simulink model "Model_Guido_v4_2020a"  (R2020a)
settings: Solver=FixedStepAuto  StartTime=0.0  StopTime=10  RelTol=1e-3
undefined symbols (not defined in the file): Bvx, Bvy, Bw, Cvx, Cvy, Cw, d, DiscIntNeverNeededParam, J, K_fsfb, K_int, Kt, l, M, r, Ti, Ts
libraries: simulink x1
settings Model: Creator=User  LastModifiedBy=User
settings SolverCC: ZeroCrossControl=EnableAll  ZeroCrossAlgorithm=Adaptive
settings DebuggingCC: IgnoredZcDiagnostic=none

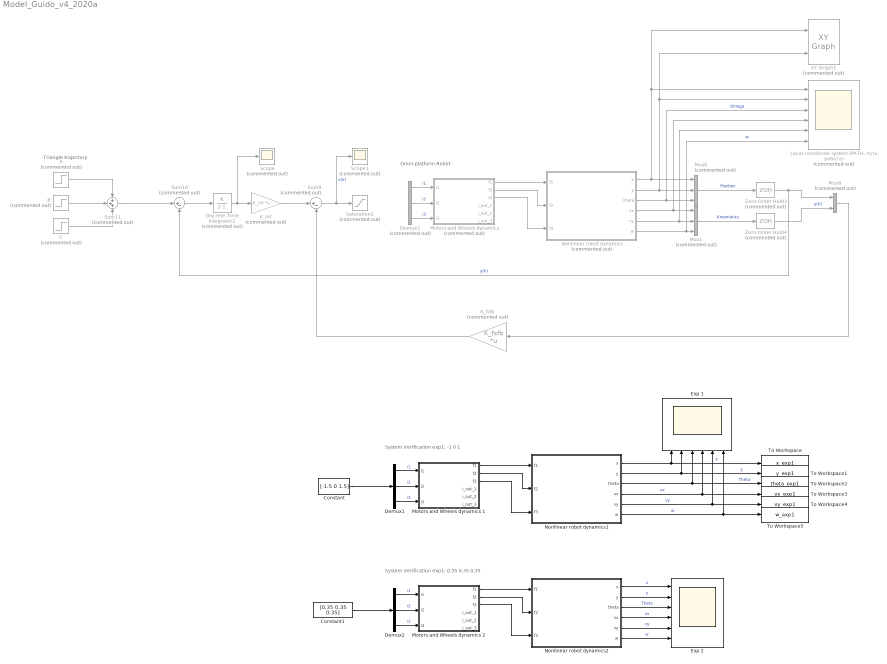
== system Model_Guido_v4_2020a ==
  note: Omni-platform Robot
  note: Triangle trajectory
  note: System Verification exp1: -1 0 1
  note: System Verification exp1: 0.35 0.35 0.35
  A : Step  Commented=on  Time=0  Before=[1 0.5 pi/2]  After=[0.5 -sqrt(3)/2 1]  SampleTime=Ts
  B : Step  Commented=on  Time=6  Before=[0 0 0]  After=[-1 0 1]  SampleTime=Ts
  C : Step  Commented=on  Time=12  Before=[0 0 0]  After=[0.5 sqrt(3)/2 0]  SampleTime=Ts
  Constant : Constant  Value=[-1.5 0 1.5]  SampleTime=0.0866
  Constant1 : Constant  Value=[0.35 0.35 0.35]  SampleTime=0.02
  Demux1 : Demux  Outputs=3
  Demux2 : Demux  Outputs=3
  Demux3 : Demux  Commented=on  Outputs=3
  Discrete-Time Integrator2 : DiscreteIntegrator  Commented=on  IntegratorMethod=Accumulation: Forward Euler  InitialCondition=[ 0 0 0]  SampleTime=Ts  ICPrevOutput=DiscIntNeverNeededParam  ICPrevScaledInput=DiscIntNeverNeededParam
  Exp 1 : Scope  NumInputPorts=6
  Exp 2 : Scope  NumInputPorts=6
  K_fsfb : Gain  Commented=on  Gain=K_fsfb  Multiplication=Matrix(K*u) (u vector)
  K_int : Gain  Commented=on  Gain=K_int  Multiplication=Matrix(K*u) (u vector)
  "Local coordinate system (PATH, путь робота)" : Scope  Commented=on  NumInputPorts=6
  "Motors and Wheels dynamics " : Subsystem  Commented=on
  Motors and Wheels dynamics 1 : Subsystem
  Motors and Wheels dynamics 2 : Subsystem
  Mux1 : Mux  Commented=on  Inputs=3
  Mux6 : Mux  Commented=on  Inputs=3
  Mux8 : Mux  Commented=on  Inputs=2
  Nonlinear robot dynamics : Subsystem  Commented=on
  Nonlinear robot dynamics1 : Subsystem
  Nonlinear robot dynamics2 : Subsystem
  Saturation2 : Saturate  Commented=on  UpperLimit=1  LowerLimit=-1
  Scope : Scope  Commented=on
  Scope1 : Scope  Commented=on
  Sum10 : Sum  Commented=on  Inputs=|+-
  Sum11 : Sum  Commented=on  Inputs=+++
  Sum9 : Sum  Commented=on  Inputs=|+-
  To Workspace : ToWorkspace  VariableName=x_exp1  SampleTime=-1
      settings: Save2DSignal=2-D array (concatenate along first dimension)
  To Workspace1 : ToWorkspace  VariableName=y_exp1  SaveFormat=Timeseries  SampleTime=-1
  To Workspace2 : ToWorkspace  VariableName=theta_exp1  SaveFormat=Timeseries  SampleTime=-1
  To Workspace3 : ToWorkspace  VariableName=vx_exp1  SaveFormat=Timeseries  SampleTime=-1
  To Workspace4 : ToWorkspace  VariableName=vy_exp1  SaveFormat=Timeseries  SampleTime=-1
  To Workspace5 : ToWorkspace  VariableName=w_exp1  SaveFormat=Timeseries  SampleTime=-1
  XY Graph1 : simulink/Sinks/XY Graph  Commented=on  xmin=-1  xmax=1  ymin=-1  ymax=1  st=-1
  Zero-Order Hold3 : ZeroOrderHold  Commented=on  SampleTime=Ts
  Zero-Order Hold4 : ZeroOrderHold  Commented=on  SampleTime=Ts
  wires:
  Nonlinear robot dynamics/1(x) -> "Local coordinate system (PATH, путь робота)"/1, XY Graph1/1, Mux6/1
  Nonlinear robot dynamics/2(y) -> "Local coordinate system (PATH, путь робота)"/2, XY Graph1/2, Mux6/2
  Nonlinear robot dynamics/3(theta) -> "Local coordinate system (PATH, путь робота)"/3, Mux6/3  "Omega"
  Mux6/1 -> Zero-Order Hold3/1  "Position"
  C/1 -> Sum11/3
  Sum9/1 -> Scope1/1, Saturation2/1  "u(k)"
  Zero-Order Hold3/1 -> Mux8/1, Sum10/2  "y(k)"
  Discrete-Time Integrator2/1 -> Scope/1, K_int/1
  Sum10/1 -> Discrete-Time Integrator2/1
  A/1 -> Sum11/1
  B/1 -> Sum11/2
  Nonlinear robot dynamics/5(vy) -> Mux1/2, "Local coordinate system (PATH, путь робота)"/5
  Nonlinear robot dynamics/6(w) -> Mux1/3, "Local coordinate system (PATH, путь робота)"/6  "w"
  Nonlinear robot dynamics/4(vx) -> Mux1/1, "Local coordinate system (PATH, путь робота)"/4
  Demux3/1 -> "Motors and Wheels dynamics "/1(i1)  "i1"
  Demux3/2 -> "Motors and Wheels dynamics "/2(i2)  "i2"
  Demux3/3 -> "Motors and Wheels dynamics "/3(i3)  "i3"
  "Motors and Wheels dynamics "/1(f1) -> Nonlinear robot dynamics/1(f1)
  "Motors and Wheels dynamics "/2(f2) -> Nonlinear robot dynamics/2(f2)
  "Motors and Wheels dynamics "/3(f3) -> Nonlinear robot dynamics/3(f3)
  Zero-Order Hold4/1 -> Mux8/2  "y(k)"
  Mux1/1 -> Zero-Order Hold4/1  "Kinematics"
  Mux8/1 -> K_fsfb/1
  K_int/1 -> Sum9/1
  K_fsfb/1 -> Sum9/2
  Sum11/1 -> Sum10/1
  Motors and Wheels dynamics 1/3(f3) -> Nonlinear robot dynamics1/3(f3)
  Demux1/2 -> Motors and Wheels dynamics 1/2(i2)  "i2"
  Demux1/3 -> Motors and Wheels dynamics 1/3(i3)  "i3"
  Motors and Wheels dynamics 1/2(f2) -> Nonlinear robot dynamics1/2(f2)
  Demux1/1 -> Motors and Wheels dynamics 1/1(i1)  "i1"
  Motors and Wheels dynamics 1/1(f1) -> Nonlinear robot dynamics1/1(f1)
  Motors and Wheels dynamics 2/3(f3) -> Nonlinear robot dynamics2/3(f3)
  Demux2/2 -> Motors and Wheels dynamics 2/2(i2)  "i2"
  Demux2/3 -> Motors and Wheels dynamics 2/3(i3)  "i3"
  Motors and Wheels dynamics 2/2(f2) -> Nonlinear robot dynamics2/2(f2)
  Demux2/1 -> Motors and Wheels dynamics 2/1(i1)  "i1"
  Motors and Wheels dynamics 2/1(f1) -> Nonlinear robot dynamics2/1(f1)
  Nonlinear robot dynamics1/1(x) -> Exp 1/1, To Workspace/1  "x"
  Nonlinear robot dynamics1/2(y) -> Exp 1/2, To Workspace1/1  "y"
  Nonlinear robot dynamics1/3(theta) -> Exp 1/3, To Workspace2/1  "Theta"
  Nonlinear robot dynamics1/4(vx) -> Exp 1/4, To Workspace3/1  "vx"
  Nonlinear robot dynamics1/5(vy) -> To Workspace4/1, Exp 1/5  "vy"
  Nonlinear robot dynamics1/6(w) -> Exp 1/6, To Workspace5/1  "w"
  Nonlinear robot dynamics2/1(x) -> Exp 2/1  "x"
  Nonlinear robot dynamics2/2(y) -> Exp 2/2  "y"
  Nonlinear robot dynamics2/3(theta) -> Exp 2/3  "Theta"
  Nonlinear robot dynamics2/4(vx) -> Exp 2/4  "vx"
  Nonlinear robot dynamics2/5(vy) -> Exp 2/5  "vy"
  Nonlinear robot dynamics2/6(w) -> Exp 2/6  "w"
  Constant1/1 -> Demux2/1
  Constant/1 -> Demux1/1

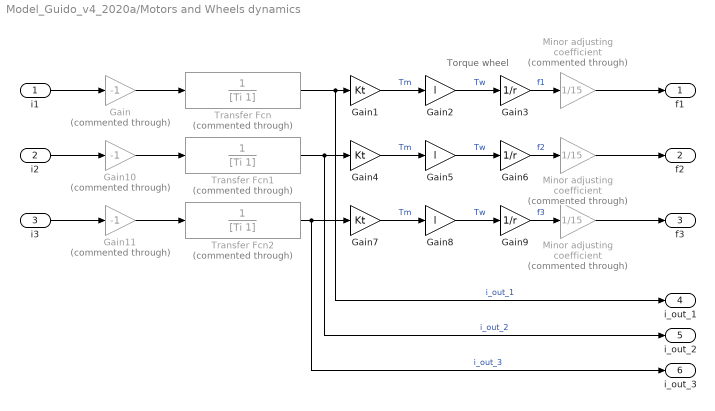
== system Model_Guido_v4_2020a/Motors and Wheels dynamics  ==
  note: Torque wheel
  i1 : Inport
  i2 : Inport  Port=2
  i3 : Inport  Port=3
  Gain : Gain  Commented=through  Gain=-1
  Gain1 : Gain  Gain=Kt
  Gain10 : Gain  Commented=through  Gain=-1
  Gain11 : Gain  Commented=through  Gain=-1
  Gain2 : Gain  Gain=l
  Gain3 : Gain  Gain=1/r
  Gain4 : Gain  Gain=Kt
  Gain5 : Gain  Gain=l
  Gain6 : Gain  Gain=1/r
  Gain7 : Gain  Gain=Kt
  Gain8 : Gain  Gain=l
  Gain9 : Gain  Gain=1/r
  "Minor adjusting coefficient  " : Gain  Commented=through  Gain=1/15
  "Minor adjusting coefficient   " : Gain  Commented=through  Gain=1/15
  "Minor adjusting coefficient    " : Gain  Commented=through  Gain=1/15
  Transfer Fcn : TransferFcn  Commented=through  Denominator=[Ti 1]
  Transfer Fcn1 : TransferFcn  Commented=through  Denominator=[Ti 1]
  Transfer Fcn2 : TransferFcn  Commented=through  Denominator=[Ti 1]
  f1 : Outport
  f2 : Outport  Port=2
  f3 : Outport  Port=3
  i_out_1 : Outport  Port=4
  i_out_2 : Outport  Port=5
  i_out_3 : Outport  Port=6
  wires:
  i2/1 -> Gain10/1
  Gain1/1 -> Gain2/1  "Tm"
  Gain8/1 -> Gain9/1  "Tw"
  Gain5/1 -> Gain6/1  "Tw"
  Transfer Fcn/1 -> i_out_1/1, Gain1/1  "i_out_1"
  Transfer Fcn2/1 -> i_out_3/1, Gain7/1  "i_out_3"
  i3/1 -> Gain11/1
  Gain2/1 -> Gain3/1  "Tw"
  Gain7/1 -> Gain8/1  "Tm"
  Transfer Fcn1/1 -> i_out_2/1, Gain4/1  "i_out_2"
  Gain4/1 -> Gain5/1  "Tm"
  Gain3/1 -> "Minor adjusting coefficient  "/1  "f1"
  Gain6/1 -> "Minor adjusting coefficient   "/1  "f2"
  i1/1 -> Gain/1
  Gain9/1 -> "Minor adjusting coefficient    "/1  "f3"
  Gain/1 -> Transfer Fcn/1
  Gain10/1 -> Transfer Fcn1/1
  Gain11/1 -> Transfer Fcn2/1
  "Minor adjusting coefficient  "/1 -> f1/1
  "Minor adjusting coefficient   "/1 -> f2/1
  "Minor adjusting coefficient    "/1 -> f3/1

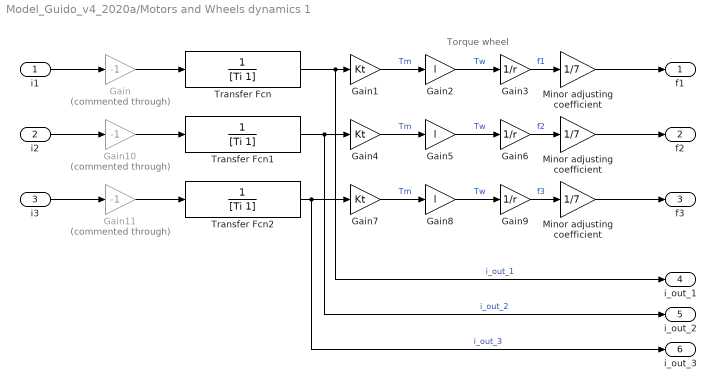
== system Model_Guido_v4_2020a/Motors and Wheels dynamics 1 ==
  note: Torque wheel
  i1 : Inport
  i2 : Inport  Port=2
  i3 : Inport  Port=3
  Gain : Gain  Commented=through  Gain=-1
  Gain1 : Gain  Gain=Kt
  Gain10 : Gain  Commented=through  Gain=-1
  Gain11 : Gain  Commented=through  Gain=-1
  Gain2 : Gain  Gain=l
  Gain3 : Gain  Gain=1/r
  Gain4 : Gain  Gain=Kt
  Gain5 : Gain  Gain=l
  Gain6 : Gain  Gain=1/r
  Gain7 : Gain  Gain=Kt
  Gain8 : Gain  Gain=l
  Gain9 : Gain  Gain=1/r
  "Minor adjusting coefficient  " : Gain  Gain=1/7
  "Minor adjusting coefficient   " : Gain  Gain=1/7
  "Minor adjusting coefficient    " : Gain  Gain=1/7
  Transfer Fcn : TransferFcn  Denominator=[Ti 1]
  Transfer Fcn1 : TransferFcn  Denominator=[Ti 1]
  Transfer Fcn2 : TransferFcn  Denominator=[Ti 1]
  f1 : Outport
  f2 : Outport  Port=2
  f3 : Outport  Port=3
  i_out_1 : Outport  Port=4
  i_out_2 : Outport  Port=5
  i_out_3 : Outport  Port=6
  wires:
  i2/1 -> Gain10/1
  Gain1/1 -> Gain2/1  "Tm"
  Gain8/1 -> Gain9/1  "Tw"
  Gain5/1 -> Gain6/1  "Tw"
  Transfer Fcn/1 -> i_out_1/1, Gain1/1  "i_out_1"
  Transfer Fcn2/1 -> i_out_3/1, Gain7/1  "i_out_3"
  i3/1 -> Gain11/1
  Gain2/1 -> Gain3/1  "Tw"
  Gain7/1 -> Gain8/1  "Tm"
  Transfer Fcn1/1 -> i_out_2/1, Gain4/1  "i_out_2"
  Gain4/1 -> Gain5/1  "Tm"
  Gain3/1 -> "Minor adjusting coefficient  "/1  "f1"
  Gain6/1 -> "Minor adjusting coefficient   "/1  "f2"
  i1/1 -> Gain/1
  Gain9/1 -> "Minor adjusting coefficient    "/1  "f3"
  Gain/1 -> Transfer Fcn/1
  Gain10/1 -> Transfer Fcn1/1
  Gain11/1 -> Transfer Fcn2/1
  "Minor adjusting coefficient  "/1 -> f1/1
  "Minor adjusting coefficient   "/1 -> f2/1
  "Minor adjusting coefficient    "/1 -> f3/1

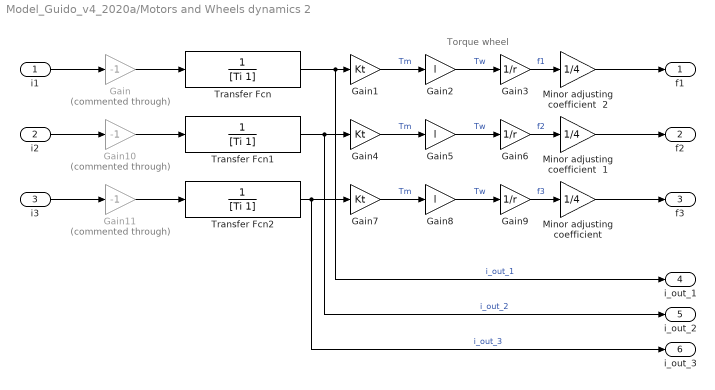
== system Model_Guido_v4_2020a/Motors and Wheels dynamics 2 ==
  note: Torque wheel
  i1 : Inport
  i2 : Inport  Port=2
  i3 : Inport  Port=3
  Gain : Gain  Commented=through  Gain=-1
  Gain1 : Gain  Gain=Kt
  Gain10 : Gain  Commented=through  Gain=-1
  Gain11 : Gain  Commented=through  Gain=-1
  Gain2 : Gain  Gain=l
  Gain3 : Gain  Gain=1/r
  Gain4 : Gain  Gain=Kt
  Gain5 : Gain  Gain=l
  Gain6 : Gain  Gain=1/r
  Gain7 : Gain  Gain=Kt
  Gain8 : Gain  Gain=l
  Gain9 : Gain  Gain=1/r
  "Minor adjusting coefficient  " : Gain  Gain=1/4
  Minor adjusting coefficient  1 : Gain  Gain=1/4
  Minor adjusting coefficient  2 : Gain  Gain=1/4
  Transfer Fcn : TransferFcn  Denominator=[Ti 1]
  Transfer Fcn1 : TransferFcn  Denominator=[Ti 1]
  Transfer Fcn2 : TransferFcn  Denominator=[Ti 1]
  f1 : Outport
  f2 : Outport  Port=2
  f3 : Outport  Port=3
  i_out_1 : Outport  Port=4
  i_out_2 : Outport  Port=5
  i_out_3 : Outport  Port=6
  wires:
  i2/1 -> Gain10/1
  Gain1/1 -> Gain2/1  "Tm"
  Gain8/1 -> Gain9/1  "Tw"
  Gain5/1 -> Gain6/1  "Tw"
  Transfer Fcn/1 -> i_out_1/1, Gain1/1  "i_out_1"
  Transfer Fcn2/1 -> i_out_3/1, Gain7/1  "i_out_3"
  i3/1 -> Gain11/1
  Gain2/1 -> Gain3/1  "Tw"
  Gain7/1 -> Gain8/1  "Tm"
  Transfer Fcn1/1 -> i_out_2/1, Gain4/1  "i_out_2"
  Gain4/1 -> Gain5/1  "Tm"
  Gain3/1 -> Minor adjusting coefficient  2/1  "f1"
  Gain6/1 -> Minor adjusting coefficient  1/1  "f2"
  i1/1 -> Gain/1
  Gain9/1 -> "Minor adjusting coefficient  "/1  "f3"
  Gain/1 -> Transfer Fcn/1
  Gain10/1 -> Transfer Fcn1/1
  Gain11/1 -> Transfer Fcn2/1
  Minor adjusting coefficient  2/1 -> f1/1
  Minor adjusting coefficient  1/1 -> f2/1
  "Minor adjusting coefficient  "/1 -> f3/1

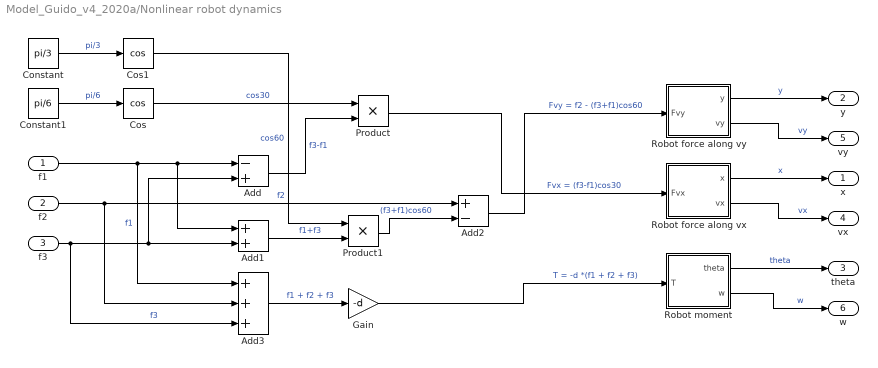
== system Model_Guido_v4_2020a/Nonlinear robot dynamics ==
  f1 : Inport
  f2 : Inport  Port=2
  f3 : Inport  Port=3
  Add : Sum  Inputs=-+
  Add1 : Sum
  Add2 : Sum  Inputs=+-
  Add3 : Sum  Inputs=+++
  Constant : Constant  Value=pi/3
  Constant1 : Constant  Value=pi/6
  Cos : Trigonometry  Operator=cos
  Cos1 : Trigonometry  Operator=cos
  Gain : Gain  Gain=-d
  Product : Product
  Product1 : Product
  Robot force along vx : Subsystem
  Robot force along vy : Subsystem
  Robot moment : Subsystem
  x : Outport
  y : Outport  Port=2
  theta : Outport  Port=3
  vx : Outport  Port=4
  vy : Outport  Port=5
  w : Outport  Port=6
  wires:
  f3/1 -> Add3/3, Add1/2, Add/2  "f3"
  f1/1 -> Add3/1, Add/1, Add1/1  "f1"
  f2/1 -> Add3/2, Add2/1  "f2"
  Robot force along vy/1(y) -> y/1  "y"
  Robot moment/1(theta) -> theta/1  "theta"
  Robot force along vx/2(vx) -> vx/1  "vx"
  Robot force along vx/1(x) -> x/1  "x"
  Robot moment/2(w) -> w/1  "w"
  Robot force along vy/2(vy) -> vy/1  "vy"
  Add/1 -> Product/2  "f3-f1"
  Constant1/1 -> Cos/1  "pi/6"
  Cos/1 -> Product/1  "cos30"
  Product/1 -> Robot force along vx/1(Fvx)  "Fvx = (f3-f1)cos30"
  Constant/1 -> Cos1/1  "pi/3"
  Cos1/1 -> Product1/1  "cos60"
  Add1/1 -> Product1/2  "f1+f3"
  Product1/1 -> Add2/2  "(f3+f1)cos60"
  Add2/1 -> Robot force along vy/1(Fvy)  "Fvy = f2 - (f3+f1)cos60"
  Add3/1 -> Gain/1  "f1 + f2 + f3"
  Gain/1 -> Robot moment/1(T)  "T = -d *(f1 + f2 + f3)"

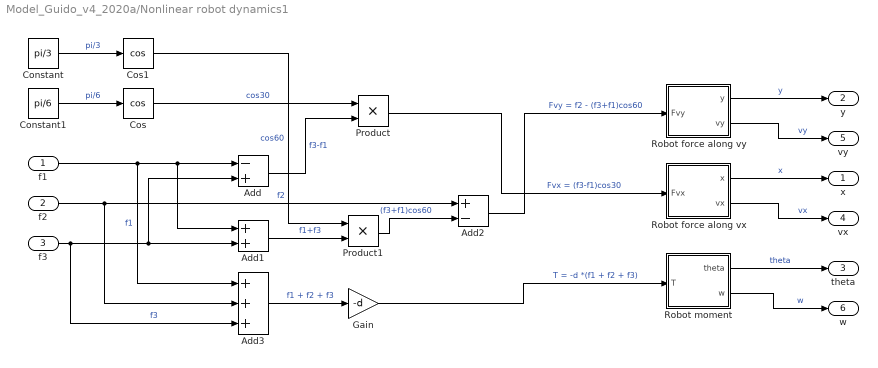
== system Model_Guido_v4_2020a/Nonlinear robot dynamics1 ==
  f1 : Inport
  f2 : Inport  Port=2
  f3 : Inport  Port=3
  Add : Sum  Inputs=-+
  Add1 : Sum
  Add2 : Sum  Inputs=+-
  Add3 : Sum  Inputs=+++
  Constant : Constant  Value=pi/3
  Constant1 : Constant  Value=pi/6
  Cos : Trigonometry  Operator=cos
  Cos1 : Trigonometry  Operator=cos
  Gain : Gain  Gain=-d
  Product : Product
  Product1 : Product
  Robot force along vx : Subsystem
  Robot force along vy : Subsystem
  Robot moment : Subsystem
  x : Outport
  y : Outport  Port=2
  theta : Outport  Port=3
  vx : Outport  Port=4
  vy : Outport  Port=5
  w : Outport  Port=6
  wires:
  f3/1 -> Add3/3, Add1/2, Add/2  "f3"
  f1/1 -> Add3/1, Add/1, Add1/1  "f1"
  f2/1 -> Add3/2, Add2/1  "f2"
  Robot force along vy/1(y) -> y/1  "y"
  Robot moment/1(theta) -> theta/1  "theta"
  Robot force along vx/2(vx) -> vx/1  "vx"
  Robot force along vx/1(x) -> x/1  "x"
  Robot moment/2(w) -> w/1  "w"
  Robot force along vy/2(vy) -> vy/1  "vy"
  Add/1 -> Product/2  "f3-f1"
  Constant1/1 -> Cos/1  "pi/6"
  Cos/1 -> Product/1  "cos30"
  Product/1 -> Robot force along vx/1(Fvx)  "Fvx = (f3-f1)cos30"
  Constant/1 -> Cos1/1  "pi/3"
  Cos1/1 -> Product1/1  "cos60"
  Add1/1 -> Product1/2  "f1+f3"
  Product1/1 -> Add2/2  "(f3+f1)cos60"
  Add2/1 -> Robot force along vy/1(Fvy)  "Fvy = f2 - (f3+f1)cos60"
  Add3/1 -> Gain/1  "f1 + f2 + f3"
  Gain/1 -> Robot moment/1(T)  "T = -d *(f1 + f2 + f3)"

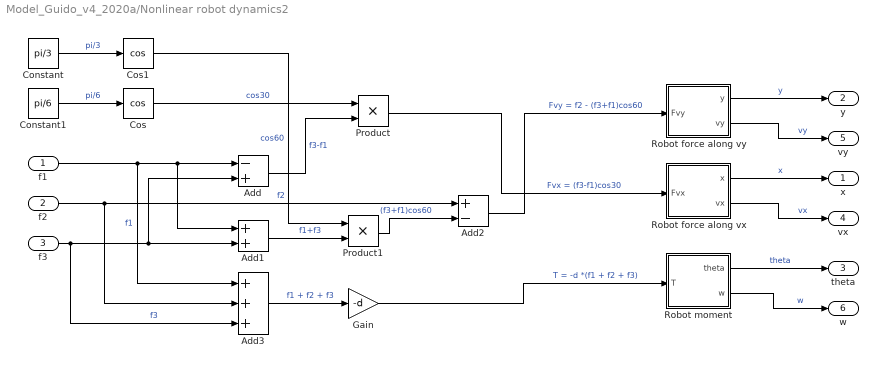
== system Model_Guido_v4_2020a/Nonlinear robot dynamics2 ==
  f1 : Inport
  f2 : Inport  Port=2
  f3 : Inport  Port=3
  Add : Sum  Inputs=-+
  Add1 : Sum
  Add2 : Sum  Inputs=+-
  Add3 : Sum  Inputs=+++
  Constant : Constant  Value=pi/3
  Constant1 : Constant  Value=pi/6
  Cos : Trigonometry  Operator=cos
  Cos1 : Trigonometry  Operator=cos
  Gain : Gain  Gain=-d
  Product : Product
  Product1 : Product
  Robot force along vx : Subsystem
  Robot force along vy : Subsystem
  Robot moment : Subsystem
  x : Outport
  y : Outport  Port=2
  theta : Outport  Port=3
  vx : Outport  Port=4
  vy : Outport  Port=5
  w : Outport  Port=6
  wires:
  f3/1 -> Add3/3, Add1/2, Add/2  "f3"
  f1/1 -> Add3/1, Add/1, Add1/1  "f1"
  f2/1 -> Add3/2, Add2/1  "f2"
  Robot force along vy/1(y) -> y/1  "y"
  Robot moment/1(theta) -> theta/1  "theta"
  Robot force along vx/2(vx) -> vx/1  "vx"
  Robot force along vx/1(x) -> x/1  "x"
  Robot moment/2(w) -> w/1  "w"
  Robot force along vy/2(vy) -> vy/1  "vy"
  Add/1 -> Product/2  "f3-f1"
  Constant1/1 -> Cos/1  "pi/6"
  Cos/1 -> Product/1  "cos30"
  Product/1 -> Robot force along vx/1(Fvx)  "Fvx = (f3-f1)cos30"
  Constant/1 -> Cos1/1  "pi/3"
  Cos1/1 -> Product1/1  "cos60"
  Add1/1 -> Product1/2  "f1+f3"
  Product1/1 -> Add2/2  "(f3+f1)cos60"
  Add2/1 -> Robot force along vy/1(Fvy)  "Fvy = f2 - (f3+f1)cos60"
  Add3/1 -> Gain/1  "f1 + f2 + f3"
  Gain/1 -> Robot moment/1(T)  "T = -d *(f1 + f2 + f3)"

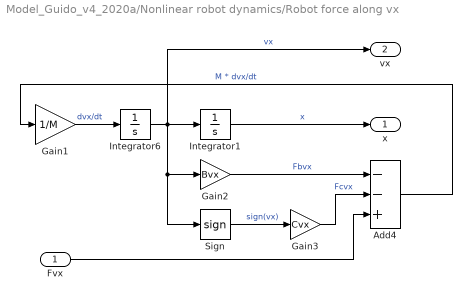
== system Model_Guido_v4_2020a/Nonlinear robot dynamics/Robot force along vx ==
  Fvx : Inport
  Add4 : Sum  Inputs=--+
  Gain1 : Gain  Gain=1/M
  Gain2 : Gain  Gain=Bvx
  Gain3 : Gain  Gain=Cvx
  Integrator1 : Integrator  ContinuousStateAttributes='x'
  Integrator6 : Integrator  ContinuousStateAttributes='vx'
  Sign : Signum
  x : Outport
  vx : Outport  Port=2
  wires:
  Fvx/1 -> Add4/3
  Sign/1 -> Gain3/1  "sign(vx)"
  Gain2/1 -> Add4/1  "Fbvx"
  Gain3/1 -> Add4/2  "Fcvx"
  Integrator1/1 -> x/1  "x"
  Integrator6/1 -> vx/1, Integrator1/1, Sign/1, Gain2/1  "vx"
  Gain1/1 -> Integrator6/1  "dvx/dt"
  Add4/1 -> Gain1/1  "M * dvx/dt"

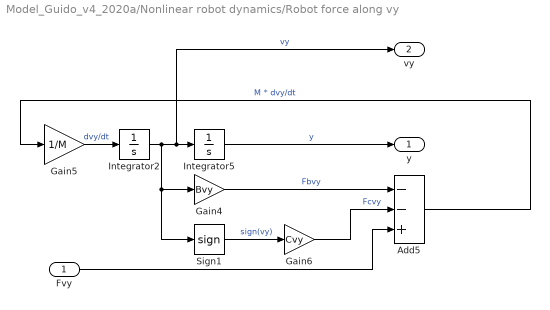
== system Model_Guido_v4_2020a/Nonlinear robot dynamics/Robot force along vy ==
  Fvy : Inport
  Add5 : Sum  Inputs=--+
  Gain4 : Gain  Gain=Bvy
  Gain5 : Gain  Gain=1/M
  Gain6 : Gain  Gain=Cvy
  Integrator2 : Integrator  ContinuousStateAttributes='vy'
  Integrator5 : Integrator  ContinuousStateAttributes='y'
  Sign1 : Signum
  y : Outport
  vy : Outport  Port=2
  wires:
  Gain5/1 -> Integrator2/1  "dvy/dt"
  Integrator2/1 -> vy/1, Integrator5/1, Sign1/1, Gain4/1  "vy"
  Gain6/1 -> Add5/2  "Fcvy"
  Fvy/1 -> Add5/3
  Add5/1 -> Gain5/1  "M * dvy/dt"
  Sign1/1 -> Gain6/1  "sign(vy)"
  Gain4/1 -> Add5/1  "Fbvy"
  Integrator5/1 -> y/1  "y"

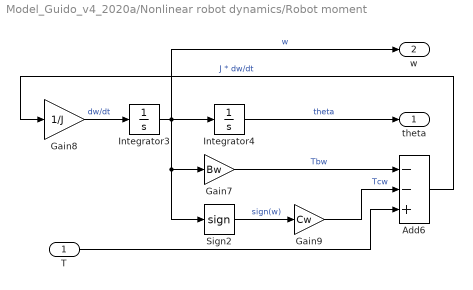
== system Model_Guido_v4_2020a/Nonlinear robot dynamics/Robot moment ==
  T : Inport
  Add6 : Sum  Inputs=--+
  Gain7 : Gain  Gain=Bw
  Gain8 : Gain  Gain=1/J
  Gain9 : Gain  Gain=Cw
  Integrator3 : Integrator  ContinuousStateAttributes='w'
  Integrator4 : Integrator  ContinuousStateAttributes='theta'
  Sign2 : Signum
  theta : Outport
  w : Outport  Port=2
  wires:
  Integrator3/1 -> w/1, Integrator4/1, Sign2/1, Gain7/1  "w"
  Gain8/1 -> Integrator3/1  "dw/dt"
  Add6/1 -> Gain8/1  "J * dw/dt"
  Gain9/1 -> Add6/2  "Tcw"
  Gain7/1 -> Add6/1  "Tbw"
  Sign2/1 -> Gain9/1  "sign(w)"
  Integrator4/1 -> theta/1  "theta"
  T/1 -> Add6/3

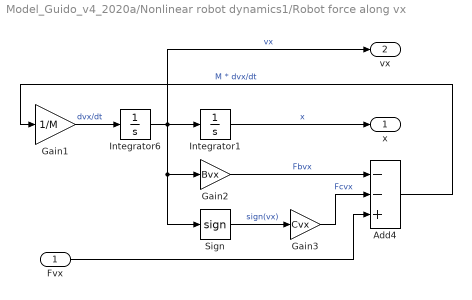
== system Model_Guido_v4_2020a/Nonlinear robot dynamics1/Robot force along vx ==
  Fvx : Inport
  Add4 : Sum  Inputs=--+
  Gain1 : Gain  Gain=1/M
  Gain2 : Gain  Gain=Bvx
  Gain3 : Gain  Gain=Cvx
  Integrator1 : Integrator  ContinuousStateAttributes='x'
  Integrator6 : Integrator  ContinuousStateAttributes='vx'
  Sign : Signum
  x : Outport
  vx : Outport  Port=2
  wires:
  Fvx/1 -> Add4/3
  Sign/1 -> Gain3/1  "sign(vx)"
  Gain2/1 -> Add4/1  "Fbvx"
  Gain3/1 -> Add4/2  "Fcvx"
  Integrator1/1 -> x/1  "x"
  Integrator6/1 -> vx/1, Integrator1/1, Sign/1, Gain2/1  "vx"
  Gain1/1 -> Integrator6/1  "dvx/dt"
  Add4/1 -> Gain1/1  "M * dvx/dt"

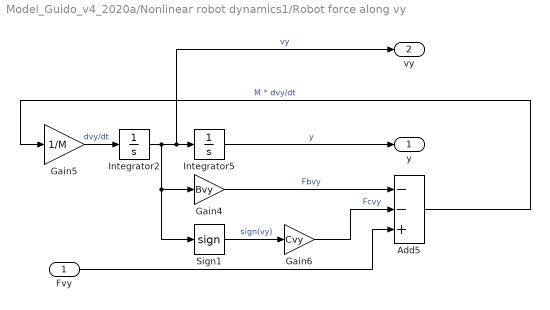
== system Model_Guido_v4_2020a/Nonlinear robot dynamics1/Robot force along vy ==
  Fvy : Inport
  Add5 : Sum  Inputs=--+
  Gain4 : Gain  Gain=Bvy
  Gain5 : Gain  Gain=1/M
  Gain6 : Gain  Gain=Cvy
  Integrator2 : Integrator  ContinuousStateAttributes='vy'
  Integrator5 : Integrator  ContinuousStateAttributes='y'
  Sign1 : Signum
  y : Outport
  vy : Outport  Port=2
  wires:
  Gain5/1 -> Integrator2/1  "dvy/dt"
  Integrator2/1 -> vy/1, Integrator5/1, Sign1/1, Gain4/1  "vy"
  Gain6/1 -> Add5/2  "Fcvy"
  Fvy/1 -> Add5/3
  Add5/1 -> Gain5/1  "M * dvy/dt"
  Sign1/1 -> Gain6/1  "sign(vy)"
  Gain4/1 -> Add5/1  "Fbvy"
  Integrator5/1 -> y/1  "y"

== system Model_Guido_v4_2020a/Nonlinear robot dynamics1/Robot moment ==
  T : Inport
  Add6 : Sum  Inputs=--+
  Gain7 : Gain  Gain=Bw
  Gain8 : Gain  Gain=1/J
  Gain9 : Gain  Gain=Cw
  Integrator3 : Integrator  ContinuousStateAttributes='w'
  Integrator4 : Integrator  ContinuousStateAttributes='theta'
  Sign2 : Signum
  theta : Outport
  w : Outport  Port=2
  wires:
  Integrator3/1 -> w/1, Integrator4/1, Sign2/1, Gain7/1  "w"
  Gain8/1 -> Integrator3/1  "dw/dt"
  Add6/1 -> Gain8/1  "J * dw/dt"
  Gain9/1 -> Add6/2  "Tcw"
  Gain7/1 -> Add6/1  "Tbw"
  Sign2/1 -> Gain9/1  "sign(w)"
  Integrator4/1 -> theta/1  "theta"
  T/1 -> Add6/3

== system Model_Guido_v4_2020a/Nonlinear robot dynamics2/Robot force along vx ==
  Fvx : Inport
  Add4 : Sum  Inputs=--+
  Gain1 : Gain  Gain=1/M
  Gain2 : Gain  Gain=Bvx
  Gain3 : Gain  Gain=Cvx
  Integrator1 : Integrator  ContinuousStateAttributes='x'
  Integrator6 : Integrator  ContinuousStateAttributes='vx'
  Sign : Signum
  x : Outport
  vx : Outport  Port=2
  wires:
  Fvx/1 -> Add4/3
  Sign/1 -> Gain3/1  "sign(vx)"
  Gain2/1 -> Add4/1  "Fbvx"
  Gain3/1 -> Add4/2  "Fcvx"
  Integrator1/1 -> x/1  "x"
  Integrator6/1 -> vx/1, Integrator1/1, Sign/1, Gain2/1  "vx"
  Gain1/1 -> Integrator6/1  "dvx/dt"
  Add4/1 -> Gain1/1  "M * dvx/dt"

== system Model_Guido_v4_2020a/Nonlinear robot dynamics2/Robot force along vy ==
  Fvy : Inport
  Add5 : Sum  Inputs=--+
  Gain4 : Gain  Gain=Bvy
  Gain5 : Gain  Gain=1/M
  Gain6 : Gain  Gain=Cvy
  Integrator2 : Integrator  ContinuousStateAttributes='vy'
  Integrator5 : Integrator  ContinuousStateAttributes='y'
  Sign1 : Signum
  y : Outport
  vy : Outport  Port=2
  wires:
  Gain5/1 -> Integrator2/1  "dvy/dt"
  Integrator2/1 -> vy/1, Integrator5/1, Sign1/1, Gain4/1  "vy"
  Gain6/1 -> Add5/2  "Fcvy"
  Fvy/1 -> Add5/3
  Add5/1 -> Gain5/1  "M * dvy/dt"
  Sign1/1 -> Gain6/1  "sign(vy)"
  Gain4/1 -> Add5/1  "Fbvy"
  Integrator5/1 -> y/1  "y"

== system Model_Guido_v4_2020a/Nonlinear robot dynamics2/Robot moment ==
  T : Inport
  Add6 : Sum  Inputs=--+
  Gain7 : Gain  Gain=Bw
  Gain8 : Gain  Gain=1/J
  Gain9 : Gain  Gain=Cw
  Integrator3 : Integrator  ContinuousStateAttributes='w'
  Integrator4 : Integrator  ContinuousStateAttributes='theta'
  Sign2 : Signum
  theta : Outport
  w : Outport  Port=2
  wires:
  Integrator3/1 -> w/1, Integrator4/1, Sign2/1, Gain7/1  "w"
  Gain8/1 -> Integrator3/1  "dw/dt"
  Add6/1 -> Gain8/1  "J * dw/dt"
  Gain9/1 -> Add6/2  "Tcw"
  Gain7/1 -> Add6/1  "Tbw"
  Sign2/1 -> Gain9/1  "sign(w)"
  Integrator4/1 -> theta/1  "theta"
  T/1 -> Add6/3
